simulink model "mcb_pmsm_foc_hall_f280049C"  (R2021b)
settings: Solver=FixedStepDiscrete  StartTime=0.0  StopTime=8  RelTol=1e-3  EnableMultiTasking=on
InitFcn:
  | position_decoder = 'hall';
  | mcb_pmsm_foc_f280049C_data;
values from neighbouring files (symbols this model uses):
  dataType = fixdt(1,32,17)    [mcb_c2000_open_loop_control_data.m]    (also in mcb_c2000_pmsm_offset_data.m; mcb_pmsm_foc_dual_f28379d_data.m = 'single'; mcb_pmsm_foc_dual_f28379d_datascript.m = 'single'; mcb_pmsm_foc_f280049C_data.m = 'single')
  inverter = mcb_SetInverterParameters('BoostXL-DRV8305')    [mcb_pmsm_foc_dual_f28379d_data.m]    (also in mcb_pmsm_foc_dual_f28379d_datascript.m; mcb_pmsm_foc_f280049C_data.m; mcb_pmsm_foc_f28335_data.m = mcb_SetInverterParameters('DRV8312-C2-KIT'); mcb_pmsm_foc_hall_f28035_data.m = mcb_SetInverterParameters('DRV8312-C2-KIT'))
  PI_params = mcb.internal.SetControllerParameters(pmsm,inverter,PU_System,T_pwm,2*Ts,Ts_speed)    [mcb_pmsm_foc_dual_f28379d_data.m]    (also in mcb_pmsm_foc_dual_f28379d_datascript.m; mcb_pmsm_foc_f280049C_data.m = mcb.internal.SetControllerParameters(pmsm,inverter,PU_System; mcb_pmsm_foc_f28335_data.m = mcb.internal.SetControllerParameters(pmsm,inverter,PU_System; mcb_pmsm_foc_hall_f28035_data.m = mcb.internal.SetControllerParameters(pmsm,inverter,PU_System)
  pmsm = struct    [c28335_pmsmfoc_data.m]    (also in mcb_pmsm_foc_dual_f28379d_data.m = mcb_SetPMSMMotorParameters('Teknic2310P'); mcb_pmsm_foc_dual_f28379d_datascript.m = mcb_SetPMSMMotorParameters('Teknic2310P'); mcb_pmsm_foc_f280049C_data.m = mcb_SetPMSMMotorParameters('BLY171D'); mcb_pmsm_foc_f28335_data.m = mcb_SetPMSMMotorParameters('BLY171D'))
  PU_System = mcb_SetPUSystem(pmsm,inverter)    [mcb_pmsm_foc_dual_f28379d_data.m]    (also in mcb_pmsm_foc_dual_f28379d_datascript.m; mcb_pmsm_foc_f280049C_data.m; mcb_pmsm_foc_f28335_data.m; mcb_pmsm_foc_hall_f28035_data.m)
  target = mcb_SetProcessorDetails('F28379D',PWM_frequency)    [mcb_pmsm_foc_dual_f28379d_data.m]    (also in mcb_pmsm_foc_dual_f28379d_datascript.m; mcb_pmsm_foc_f280049C_data.m = mcb_SetProcessorDetails('F280049C',PWM_frequency); mcb_pmsm_foc_f28335_data.m = mcb_SetProcessorDetails('F28335',PWM_frequency); mcb_pmsm_foc_hall_f28035_data.m = mcb_SetProcessorDetails('F28035',PWM_frequency))
  Ts = 5e-8    (= 5e-08)    [DCDC_Buck_Param.m]    (also in mcb_c2000_open_loop_control_data.m = T_pwm; mcb_c2000_pmsm_offset_data.m = T_pwm; mcb_pmsm_foc_dual_f28379d_data.m = 5e-05; mcb_pmsm_foc_dual_f28379d_datascript.m = 5e-05)
  Ts_motor = T_pwm/2    (= 2.5e-05)    [mcb_pmsm_foc_dual_f28379d_data.m]    (also in mcb_pmsm_foc_dual_f28379d_datascript.m; mcb_pmsm_foc_f280049C_data.m; mcb_pmsm_foc_f28335_data.m; mcb_pmsm_foc_hall_f28035_data.m)
  Ts_simulink = T_pwm/2    (= 2.5e-05)    [mcb_pmsm_foc_dual_f28379d_data.m]    (also in mcb_pmsm_foc_dual_f28379d_datascript.m; mcb_pmsm_foc_f280049C_data.m; mcb_pmsm_foc_f28335_data.m; mcb_pmsm_foc_hall_f28035_data.m)
undefined symbols (not defined in the file or in its folder): Down, GPTRIP1SEL, GPTRIP2SEL, TZ1, TZ2, Up
libraries: simulink x32, idelinklib_common x8, mcbpositiondecoderlib x7, c280xlib x7, c2802xlib x7, c28004xlib x3, mcbcontrolslib x2, demo_controls x1, c2000lib x1, mcbplantlib x1, autolibpmsmexterior x1
(part 3 of 3)

== system mcb_pmsm_foc_hall_f280049C/Embedded Processor/Hall Algorithm/Input Scaling/Read_Sensor (codegen)/Calculate Position from Hall/Atomic Hall Reading/Function-Call Subsystem ==
  function : TriggerPort  TriggerType=function-call  VariantControl=Variant
  Read Halls : Subsystem  mask(Hall sensor reader){sample_time=-1}
      mask prompts: sample_time "Sample time:"
      mask help:
      | This block outputs the state of the 3 hall sensors placed on GPIO35, 37 and 59 of LaunchXL-F280049C board.
      |
      | 0 --> GPIO59 = 0, GPIO37 = 0, GPIO35 = 0
      | 1 --> GPIO59 = 0, GPIO37 = 0, GPIO35 = 1
      | 2 --> GPIO59 = 0, GPIO37 = 1, GPIO35 = 0
      | 3 --> GPIO59 = 0, GPIO37 = 1, GPIO35 = 1
      | 4 --> GPIO59 = 1, GPIO37 = 0, GPIO35 = 0
      | 5 --> GPIO59 = 1, GPIO37 = 0, GPIO35 = 1
      | 6 --> GPIO59 = 1, GPIO37 = 1, GPIO35 = 0
      | 7 --> GPIO59 = 1, GPIO37 = 1, GPIO35 = 1
  HallSignal : Outport
  wires:
  Read Halls/1(Halls) -> HallSignal/1

== system mcb_pmsm_foc_hall_f280049C/Embedded Processor/Hall Algorithm/Input Scaling/Read_Sensor (codegen)/Calculate Position from Hall/Atomic Hall Reading/Function-Call Subsystem1 ==
  function : TriggerPort  TriggerType=function-call  VariantControl=Variant
  Memory Copy : idelinklib_common/Memory Copy  copyFrom=Specified source code symbol  copyFromAddressSource=Specify via dialog  copyFromAddress=hex2dec('00001000')  copyFromSrcCode=&ECap1Regs.TSCTR  dataTypeFrom=uint32  dataDimensionFrom=1  useOffsetFrom=off  offsetFromSrc=Specify via dialog  offsetFrom=0  strideFrom=1  copyTo=Output port  copyToAddressSource=Specify via dialog  copyToAddress=hex2dec('00002000')  copyToSrcCode=myVariableDst  dataTypeTo=uint32  useOffsetTo=off  offsetToSrc=Specify via dialog  offsetTo=0  strideTo=1  sampleTime=-1  useInitValue=off  initValueSrc=Specify constant value  initValue=1  initValueSrcCode=myInitValueVariable  useAsMask=off  maskOperator=bitwise AND  useTermValue=off  termValue=1  isRealtimeEnabled=off  emitCCBeforeWrite=off  CCBeforeWrite=/* Custom Code Before Write*/  emitCCAfterWrite=off  CCAfterWrite=/* Custom Code After Write*/  useDMACopy=off  enableBlockingMode=off
      settings: SourceProductBaseCode=ME
  Memory Copy1 : idelinklib_common/Memory Copy  copyFrom=Specified source code symbol  copyFromAddressSource=Specify via dialog  copyFromAddress=hex2dec('00001000')  copyFromSrcCode=&ECap2Regs.TSCTR  dataTypeFrom=uint32  dataDimensionFrom=1  useOffsetFrom=off  offsetFromSrc=Specify via dialog  offsetFrom=0  strideFrom=1  copyTo=Output port  copyToAddressSource=Specify via dialog  copyToAddress=hex2dec('00002000')  copyToSrcCode=myVariableDst  dataTypeTo=uint32  useOffsetTo=off  offsetToSrc=Specify via dialog  offsetTo=0  strideTo=1  sampleTime=-1  useInitValue=off  initValueSrc=Specify constant value  initValue=1  initValueSrcCode=myInitValueVariable  useAsMask=off  maskOperator=bitwise AND  useTermValue=off  termValue=1  isRealtimeEnabled=off  emitCCBeforeWrite=off  CCBeforeWrite=/* Custom Code Before Write*/  emitCCAfterWrite=off  CCAfterWrite=/* Custom Code After Write*/  useDMACopy=off  enableBlockingMode=off
      settings: SourceProductBaseCode=ME
  Memory Copy2 : idelinklib_common/Memory Copy  copyFrom=Specified source code symbol  copyFromAddressSource=Specify via dialog  copyFromAddress=hex2dec('00001000')  copyFromSrcCode=&ECap3Regs.TSCTR  dataTypeFrom=uint32  dataDimensionFrom=1  useOffsetFrom=off  offsetFromSrc=Specify via dialog  offsetFrom=0  strideFrom=1  copyTo=Output port  copyToAddressSource=Specify via dialog  copyToAddress=hex2dec('00002000')  copyToSrcCode=myVariableDst  dataTypeTo=uint32  useOffsetTo=off  offsetToSrc=Specify via dialog  offsetTo=0  strideTo=1  sampleTime=-1  useInitValue=off  initValueSrc=Specify constant value  initValue=1  initValueSrcCode=myInitValueVariable  useAsMask=off  maskOperator=bitwise AND  useTermValue=off  termValue=1  isRealtimeEnabled=off  emitCCBeforeWrite=off  CCBeforeWrite=/* Custom Code Before Write*/  emitCCAfterWrite=off  CCAfterWrite=/* Custom Code After Write*/  useDMACopy=off  enableBlockingMode=off
      settings: SourceProductBaseCode=ME
  Min : MinMax  Inputs=3
  u : Outport
  wires:
  Min/1 -> u/1
  Memory Copy2/1 -> Min/3
  Memory Copy/1 -> Min/1
  Memory Copy1/1 -> Min/2

== system mcb_pmsm_foc_hall_f280049C/Embedded Processor/Hall Algorithm/Input Scaling/Read_Sensor (codegen)/Calculate Position from Hall/Atomic Hall Reading/Integrity_Check ==
  HallSignal : Inport
  CounterIn : Inport  Port=2
  Compare To Constant : simulink/Logic and Bit Operations/Compare To Constant  relop=<  const=Ts*target.CPU_frequency*0.5  OutDataTypeStr=uint8
  If : If  IfExpression=u1 == 0
  Merge : Merge
  NOT : Logic  IconShape=distinctive  AllPortsSameDT=off  OutDataTypeStr=boolean
  No_Integrity_issue : Subsystem  TreatAsAtomicUnit=on
  Refresh_Halls : Subsystem  TreatAsAtomicUnit=on
  Relational Operator : RelationalOperator  Operator===  OutDataTypeStr=boolean  RndMeth=Simplest
  Unit Delay : UnitDelay  SampleTime=-1  HasFrameUpgradeWarning=on
  Halls : Outport
  wires:
  Refresh_Halls/1(Out1) -> Merge/2
  HallSignal/1 -> Relational Operator/1, No_Integrity_issue/1(Counter), Unit Delay/1
  If/2 -> Refresh_Halls/Action
  Merge/1 -> Halls/1
  No_Integrity_issue/1(Out1) -> Merge/1
  If/1 -> No_Integrity_issue/Action
  CounterIn/1 -> Compare To Constant/1
  Compare To Constant/1 -> NOT/2
  Relational Operator/1 -> NOT/1
  NOT/1 -> If/1
  Unit Delay/1 -> Relational Operator/2

== system mcb_pmsm_foc_hall_f280049C/Embedded Processor/Hall Algorithm/Input Scaling/Read_Sensor (codegen)/Convert ADC value to PU/Data_Type/Data_Type_Fixed_Point ==
  In1 : Inport
  Data Type Conversion : DataTypeConversion  OutDataTypeStr=fixdt(1,32,17)  ConvertRealWorld=Stored Integer (SI)  RndMeth=Simplest
  Data Type Conversion1 : DataTypeConversion  OutDataTypeStr=dataType  RndMeth=Simplest
  Q17 per unit conversion : ArithShift  BitShiftNumber=-6
  Iab_meas_PU : Outport
  wires:
  In1/1 -> Q17 per unit conversion/1
  Data Type Conversion1/1 -> Iab_meas_PU/1
  Data Type Conversion/1 -> Data Type Conversion1/1
  Q17 per unit conversion/1 -> Data Type Conversion/1

== system mcb_pmsm_foc_hall_f280049C/Embedded Processor/Hall Algorithm/Input Scaling/Read_Sensor (codegen)/Convert ADC value to PU/Data_Type/Data_Type_Float ==
  In1 : Inport
  Get ADC Voltage : Gain  Gain=target.ADC_Vref /target.ADC_MaxCount  OutDataTypeStr=dataType  RndMeth=Simplest
  Get Currents : Gain  Gain=1/inverter.ISenseVoltPerAmp  RndMeth=Simplest  OutDataTypeStr=Inherit: Same as input
  PU_Conversion : Gain  Gain=1/PU_System.I_base  RndMeth=Simplest  OutDataTypeStr=Inherit: Same as input
  Iab_meas_PU : Outport
  wires:
  Get Currents/1 -> PU_Conversion/1
  PU_Conversion/1 -> Iab_meas_PU/1
  Get ADC Voltage/1 -> Get Currents/1
  In1/1 -> Get ADC Voltage/1

== system mcb_pmsm_foc_hall_f280049C/Embedded Processor/Hall Algorithm/Input Scaling/Read_Sensor (codegen)/Calculate Position from Hall/Atomic Hall Reading/Function-Call Subsystem/Read Halls ==
  note: GPIO 35
  note: GPIO 37
  note: GPIO 59
  Bitwise Operator2 : simulink/Logic and Bit Operations/Bitwise Operator  logicop=OR  UseBitMask=off  NumInputPorts=3  BitMask=hex2dec('07000000')  BitMaskRealWorld=Stored Integer
  Hall_A : simulink/Logic and Bit Operations/Bitwise Operator  logicop=AND  UseBitMask=on  BitMask=hex2dec('00000008')  BitMaskRealWorld=Stored Integer
  Hall_B : simulink/Logic and Bit Operations/Bitwise Operator  logicop=AND  UseBitMask=on  BitMask=hex2dec('00000020')  BitMaskRealWorld=Stored Integer
  Hall_C : simulink/Logic and Bit Operations/Bitwise Operator  logicop=AND  UseBitMask=on  BitMask=hex2dec('08000000')  BitMaskRealWorld=Stored Integer
  Read GPIO DAT register : idelinklib_common/Memory Copy  copyFrom=Specified source code symbol  copyFromAddressSource=Specify via dialog  copyFromAddress=hex2dec('6FC1')  copyFromSrcCode=&GpioDataRegs.GPBDAT.all  dataTypeFrom=uint32  dataDimensionFrom=1  useOffsetFrom=off  offsetFromSrc=Specify via dialog  offsetFrom=0  strideFrom=1  copyTo=Output port  copyToAddressSource=Specify via dialog  copyToAddress=hex2dec('00002000')  copyToSrcCode=GpioDataRegs.GPADAT.bit.GPIO24  dataTypeTo=uint32  useOffsetTo=off  offsetToSrc=Specify via dialog  offsetTo=0  strideTo=1  sampleTime=-1  useInitValue=off  initValueSrc=Specify constant value  initValue=1  initValueSrcCode=myInitValueVariable  useAsMask=off  maskOperator=bitwise AND  useTermValue=off  termValue=1  isRealtimeEnabled=off  emitCCBeforeWrite=off  CCBeforeWrite=/* Custom Code Before Write*/  emitCCAfterWrite=off  CCAfterWrite=/* Custom Code After Write*/  useDMACopy=off  enableBlockingMode=off
      settings: SourceProductBaseCode=ME
  Shift Arithmetic : ArithShift  BitShiftNumber=25
  Shift Arithmetic1 : ArithShift  BitShiftNumber=4
  Shift Arithmetic2 : ArithShift  BitShiftNumber=3
  Halls : Outport
  wires:
  Hall_C/1 -> Shift Arithmetic/1
  Hall_A/1 -> Shift Arithmetic2/1
  Read GPIO DAT register/1 -> Hall_C/1, Hall_A/1, Hall_B/1
  Hall_B/1 -> Shift Arithmetic1/1
  Bitwise Operator2/1 -> Halls/1
  Shift Arithmetic/1 -> Bitwise Operator2/1
  Shift Arithmetic1/1 -> Bitwise Operator2/2
  Shift Arithmetic2/1 -> Bitwise Operator2/3

== system mcb_pmsm_foc_hall_f280049C/Embedded Processor/Hall Algorithm/Input Scaling/Read_Sensor (codegen)/Calculate Position from Hall/Atomic Hall Reading/Integrity_Check/No_Integrity_issue ==
  Counter : Inport
  Action Port : ActionPort  ActionPortLabel=if(u1 == 0)
  Out1 : Outport
  wires:
  Counter/1 -> Out1/1

== system mcb_pmsm_foc_hall_f280049C/Embedded Processor/Hall Algorithm/Input Scaling/Read_Sensor (codegen)/Calculate Position from Hall/Atomic Hall Reading/Integrity_Check/Refresh_Halls ==
  Action Port : ActionPort  ActionPortLabel=else
  Read Halls : Subsystem  mask(Hall sensor reader){sample_time=-1}
      mask prompts: sample_time "Sample time:"
      mask help:
      | This block outputs the state of the 3 hall sensors placed on GPIO35, 37 and 59 of LaunchXL-F280049C board.
      |
      | 0 --> GPIO59 = 0, GPIO37 = 0, GPIO35 = 0
      | 1 --> GPIO59 = 0, GPIO37 = 0, GPIO35 = 1
      | 2 --> GPIO59 = 0, GPIO37 = 1, GPIO35 = 0
      | 3 --> GPIO59 = 0, GPIO37 = 1, GPIO35 = 1
      | 4 --> GPIO59 = 1, GPIO37 = 0, GPIO35 = 0
      | 5 --> GPIO59 = 1, GPIO37 = 0, GPIO35 = 1
      | 6 --> GPIO59 = 1, GPIO37 = 1, GPIO35 = 0
      | 7 --> GPIO59 = 1, GPIO37 = 1, GPIO35 = 1
  Out1 : Outport
  wires:
  Read Halls/1(Halls) -> Out1/1

== system mcb_pmsm_foc_hall_f280049C/Embedded Processor/Hall Algorithm/Input Scaling/Read_Sensor (codegen)/Calculate Position from Hall/Atomic Hall Reading/Integrity_Check/Refresh_Halls/Read Halls ==
  note: GPIO 35
  note: GPIO 37
  note: GPIO 59
  Bitwise Operator2 : simulink/Logic and Bit Operations/Bitwise Operator  logicop=OR  UseBitMask=off  NumInputPorts=3  BitMask=hex2dec('07000000')  BitMaskRealWorld=Stored Integer
  Hall_A : simulink/Logic and Bit Operations/Bitwise Operator  logicop=AND  UseBitMask=on  BitMask=hex2dec('00000008')  BitMaskRealWorld=Stored Integer
  Hall_B : simulink/Logic and Bit Operations/Bitwise Operator  logicop=AND  UseBitMask=on  BitMask=hex2dec('00000020')  BitMaskRealWorld=Stored Integer
  Hall_C : simulink/Logic and Bit Operations/Bitwise Operator  logicop=AND  UseBitMask=on  BitMask=hex2dec('08000000')  BitMaskRealWorld=Stored Integer
  Read GPIO DAT register : idelinklib_common/Memory Copy  copyFrom=Specified source code symbol  copyFromAddressSource=Specify via dialog  copyFromAddress=hex2dec('6FC1')  copyFromSrcCode=&GpioDataRegs.GPBDAT.all  dataTypeFrom=uint32  dataDimensionFrom=1  useOffsetFrom=off  offsetFromSrc=Specify via dialog  offsetFrom=0  strideFrom=1  copyTo=Output port  copyToAddressSource=Specify via dialog  copyToAddress=hex2dec('00002000')  copyToSrcCode=GpioDataRegs.GPADAT.bit.GPIO24  dataTypeTo=uint32  useOffsetTo=off  offsetToSrc=Specify via dialog  offsetTo=0  strideTo=1  sampleTime=-1  useInitValue=off  initValueSrc=Specify constant value  initValue=1  initValueSrcCode=myInitValueVariable  useAsMask=off  maskOperator=bitwise AND  useTermValue=off  termValue=1  isRealtimeEnabled=off  emitCCBeforeWrite=off  CCBeforeWrite=/* Custom Code Before Write*/  emitCCAfterWrite=off  CCAfterWrite=/* Custom Code After Write*/  useDMACopy=off  enableBlockingMode=off
      settings: SourceProductBaseCode=ME
  Shift Arithmetic : ArithShift  BitShiftNumber=25
  Shift Arithmetic1 : ArithShift  BitShiftNumber=4
  Shift Arithmetic2 : ArithShift  BitShiftNumber=3
  Halls : Outport
  wires:
  Hall_C/1 -> Shift Arithmetic/1
  Hall_A/1 -> Shift Arithmetic2/1
  Read GPIO DAT register/1 -> Hall_C/1, Hall_A/1, Hall_B/1
  Hall_B/1 -> Shift Arithmetic1/1
  Bitwise Operator2/1 -> Halls/1
  Shift Arithmetic/1 -> Bitwise Operator2/1
  Shift Arithmetic1/1 -> Bitwise Operator2/2
  Shift Arithmetic2/1 -> Bitwise Operator2/3
